simulink model "OES_rel"  (R2018b)
settings: configuration reference "Configuration" (kept outside this file)
undefined symbols (not defined in the file): sats, TimeStep
settings Model: Creator=Ethan  LastModifiedBy=Ethan
settings ConfigSetRef: SourceLocation=Base Workspace

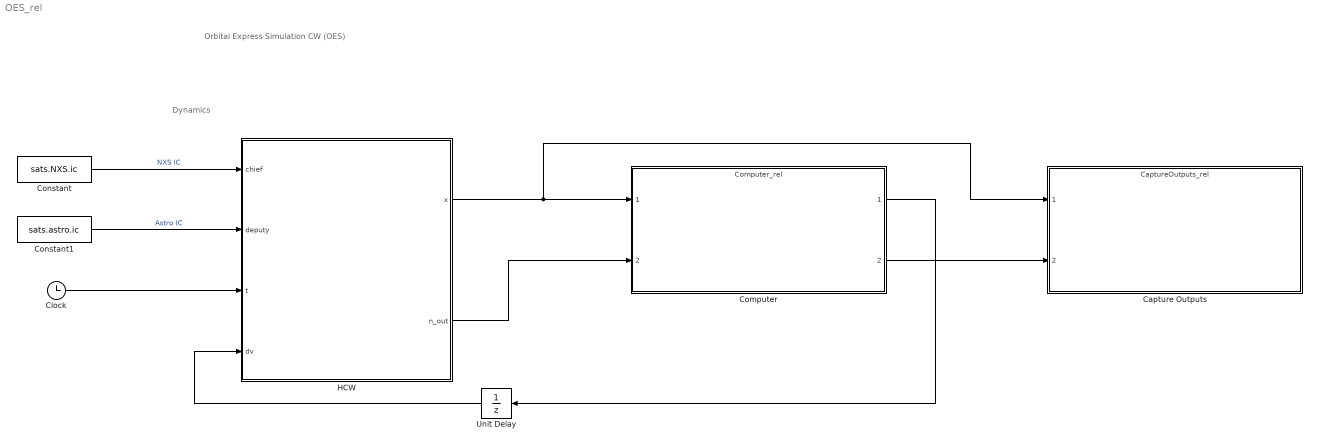
== system OES_rel ==
  note: Dynamics
  note: Orbital Express Simulation CW (OES)
  Capture Outputs : ModelReference  ModelNameDialog=CaptureOutputs_rel.slx  ParameterArgumentNames=CON  ParameterArgumentValues=CON  UsingDefaultArgumentValue=0  SimulationMode=Normal  ModelReferenceVersion=1.57
  Clock : Clock
  Computer : ModelReference  ModelNameDialog=Computer_rel.slx  ParameterArgumentNames=CON  ParameterArgumentValues=CON  UsingDefaultArgumentValue=0  SimulationMode=Normal  ModelReferenceVersion=1.233
  Constant : Constant  Value=sats.NXS.ic  OutDataTypeStr=Bus: Bus_state
  Constant1 : Constant  Value=sats.astro.ic  OutDataTypeStr=Bus: Bus_state
  HCW : MATLAB Function  TreatAsAtomicUnit=on  SystemSampleTime=TimeStep
  Unit Delay : UnitDelay  SampleTime=-1
  wires:
  Constant/1 -> HCW/1(chief)  "NXS IC"
  Constant1/1 -> HCW/2(deputy)  "Astro IC"
  Clock/1 -> HCW/3(t)
  HCW/1(x) -> Capture Outputs/1, Computer/1
  HCW/2(n_out) -> Computer/2
  Computer/2 -> Capture Outputs/2
  Computer/1 -> Unit Delay/1
  Unit Delay/1 -> HCW/4(dv)

== matlab function OES_rel/HCW ==
  data: chief input; x output; deputy input; t input; dv input; CON parameter; n_out output
function [x, n_out] = CW_prop(chief, deputy, t, dv,CON)
persistent x0 n t0 x_prev
if isempty(x0)
    [rHill,vHill] = ECI2Hill_Vectorized(chief.r_i,chief.v_i, ...
        deputy.r_i,deputy.v_i);
%     [T,~,~] = ECI2RSW(chief.r_i,chief.v_i);
%     rHill = T * (deputy.r_i - chief.r_i);
%     omega = cross(chief.r_i, chief.v_i) / norm(chief.r_i)^2;
%     dv = deputy.v_i - chief.v_i - cross(omega, rHill);
%     vHill = T * dv;
%     x0 = [rHill; vHill];
%     a0 = rvECI2oe(chief.r_i, chief.v_i, CON.mu);
    a0 = 7642;
    x0 = [.100, .010, .010, 0.0001, 0.0001, 0.0001]';
    n = sqrt(CON.mu / a0^3);
    t0 = t;
    x_prev = x0;
end

A = cw_state_matrix(n, t-t0);
n_out = n;

if any(dv ~= zeros(3, 1))
    x0(4:6) = x_prev(4:6) + dv;
    x0(1:3) = x_prev(1:3);
    A = cw_state_matrix(n, 0);
    x = A * x0;
    t0 = t;
else
    x = A * x0;
end
x_prev = x;
end
